simulink model "test"  (R2018b)
settings: Solver=FixedStepAuto  StartTime=0.0  StopTime=3  FixedStep=0.0001  RelTol=1e-3
settings Model: Creator=User  LastModifiedBy=User

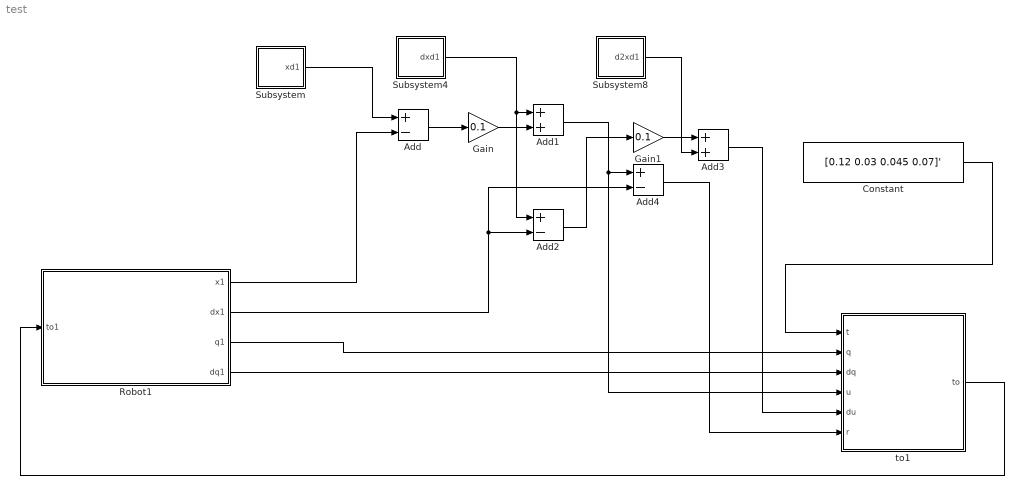
== system test ==
  Add : Sum  Inputs=+-
  Add1 : Sum
  Add2 : Sum  Inputs=+-
  Add3 : Sum
  Add4 : Sum  Inputs=+-
  Constant : Constant  Value=[0.12 0.03 0.045 0.07]'
  Gain : Gain  Gain=0.1
  Gain1 : Gain  Gain=0.1
  Robot1 : Subsystem
  Subsystem : Subsystem
  Subsystem4 : Subsystem
  Subsystem8 : Subsystem
  to1 : MATLAB Function  TreatAsAtomicUnit=on
  wires:
  to1/1(to) -> Robot1/1(to1)
  Add3/1 -> to1/5(du)
  Subsystem/1(xd1) -> Add/1
  Gain1/1 -> Add3/1
  Robot1/2(dx1) -> Add2/2, Add4/2
  Add1/1 -> to1/4(u), Add4/1
  Robot1/1(x1) -> Add/2
  Add2/1 -> Gain1/1
  Add/1 -> Gain/1
  Subsystem4/1(dxd1) -> Add2/1, Add1/1
  Add4/1 -> to1/6(r)
  Subsystem8/1(d2xd1) -> Add3/2
  Gain/1 -> Add1/2
  Robot1/3(q1) -> to1/2(q)
  Robot1/4(dq1) -> to1/3(dq)
  Constant/1 -> to1/1(t)

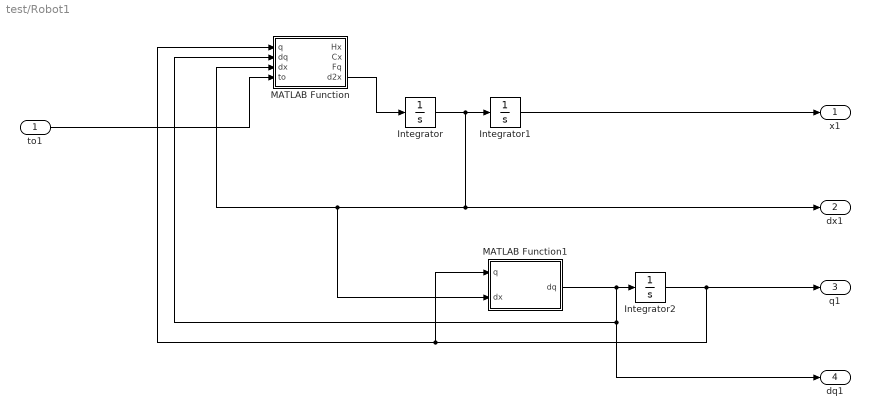
== system test/Robot1 ==
  to1 : Inport
  Integrator : Integrator  InitialCondition=[0;0]
  Integrator1 : Integrator  InitialCondition=[-3;-2]
  Integrator2 : Integrator  InitialCondition=[pi/6;pi/6]
  MATLAB Function : MATLAB Function  TreatAsAtomicUnit=on
  MATLAB Function1 : MATLAB Function  TreatAsAtomicUnit=on
  x1 : Outport
  dx1 : Outport  Port=2
  q1 : Outport  Port=3
  dq1 : Outport  Port=4
  wires:
  Integrator/1 -> MATLAB Function1/2(dx), MATLAB Function/3(dx), dx1/1, Integrator1/1
  MATLAB Function/4(d2x) -> Integrator/1
  to1/1 -> MATLAB Function/4(to)
  Integrator1/1 -> x1/1
  MATLAB Function1/1(dq) -> dq1/1, MATLAB Function/2(dq), Integrator2/1
  Integrator2/1 -> MATLAB Function/1(q), MATLAB Function1/1(q), q1/1

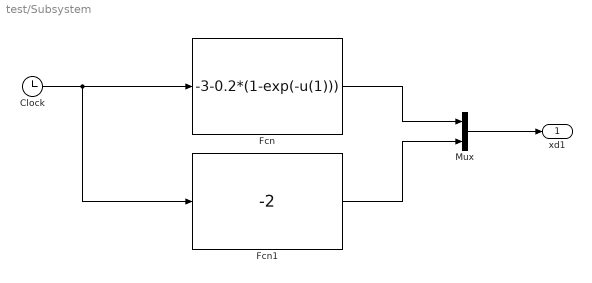
== system test/Subsystem ==
  Clock : Clock
  Fcn : Fcn  Expr=-3-0.2*(1-exp(-u(1)))
  Fcn1 : Fcn  Expr=-2
  Mux : Mux  Inputs=2
  xd1 : Outport
  wires:
  Clock/1 -> Fcn1/1, Fcn/1
  Fcn/1 -> Mux/1
  Fcn1/1 -> Mux/2
  Mux/1 -> xd1/1

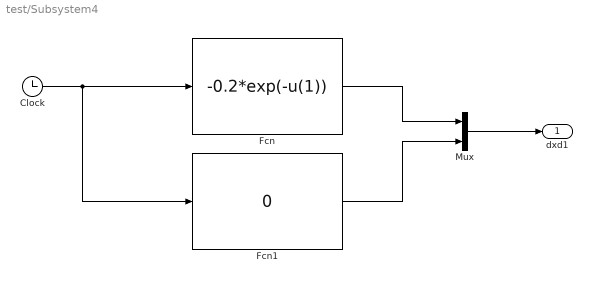
== system test/Subsystem4 ==
  Clock : Clock
  Fcn : Fcn  Expr=-0.2*exp(-u(1))
  Fcn1 : Fcn  Expr=0
  Mux : Mux  Inputs=2
  dxd1 : Outport
  wires:
  Mux/1 -> dxd1/1
  Fcn1/1 -> Mux/2
  Fcn/1 -> Mux/1
  Clock/1 -> Fcn/1, Fcn1/1

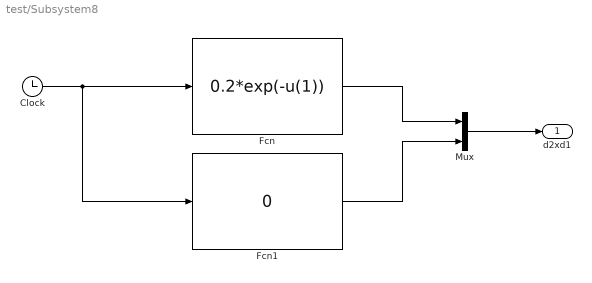
== system test/Subsystem8 ==
  Clock : Clock
  Fcn : Fcn  Expr=0.2*exp(-u(1))
  Fcn1 : Fcn  Expr=0
  Mux : Mux  Inputs=2
  d2xd1 : Outport
  wires:
  Clock/1 -> Fcn1/1, Fcn/1
  Fcn/1 -> Mux/1
  Fcn1/1 -> Mux/2
  Mux/1 -> d2xd1/1

== matlab function test/Robot1/MATLAB Function ==
  data: Hx output; Cx output; Fq output; q input; d2x output; dq input; dx input; to input
function [Hx,Cx,Fq,d2x] = fcn(q,dq,dx,to)
m1=1;
m2=1;
l1=0.3;
l2=0.3;
t1=1/3*m1*l1^2+m2*l1^2;
t2=1/3*m2*l2^2;
t3=1/2*m2*l1*l2;
t4=0.07;
q1=q(1);
q2=q(2);
Hq=[t1+t2+2*t3*cos(q2) t2+t3*cos(q2);
    t2+t3*cos(q2) t2];
dq1=dq(1);
dq2=dq(2);
Cq=[-dq2*t3*sin(q2) -(dq1+dq2)*t3*sin(q2);
    dq1*t3*sin(q2) 0];
Fq=[t4*dq1;t4*dq2];
J=[-0.3*sin(q1)-0.3*sin(q1+q2) -0.3*sin(q1+q2);
    0.3*cos(q1)+0.3*cos(q1+q2) 0.3*cos(q1+q2)];
dJ=[-0.3*dq1*cos(q1)-0.3*(dq1+dq2)*cos(q1+q2) -0.3*(dq1+dq2)*cos(q1+q2);
    -0.3*dq1*sin(q1)-0.3*(dq1+dq2)*sin(q1+q2) -0.3*(dq1+dq2)*sin(q1+q2)];
Hx=Hq*pinv(J);
Cx=Cq*pinv(J)-Hq*pinv(J)*dJ*pinv(J);
d2x=Hx\(to-Cx*dx-Fq);
end

== matlab function test/Robot1/MATLAB Function1 ==
  data: q input; dq output; dx input
function dq = fcn(q,dx)
q1=q(1);
q2=q(2);
J=[-0.3*sin(q1)-0.3*sin(q1+q2) -0.3*sin(q1+q2);
    0.3*cos(q1)+0.3*cos(q1+q2) 0.3*cos(q1+q2)];
dq=pinv(J)*dx;
end

== matlab function test/to1 ==
  data: t input; q input; dq input; u input; to output; du input; r input
function to = fcn(t,q,dq,u,du,r)
t1=t(1);
t2=t(2);
t3=t(3);
t4=t(4);
q1=q(1);
q2=q(2);
Hq=[t1+t2+2*t3*cos(q2) t2+t3*cos(q2);
    t2+t3*cos(q2) t2];
dq1=dq(1);
dq2=dq(2);
Cq=[-dq2*t3*sin(q2) -(dq1+dq2)*t3*sin(q2);
    dq1*t3*sin(q2) 0];
Fq=[t4*dq1;t4*dq2];
J=[-0.3*sin(q1)-0.3*sin(q1+q2) -0.3*sin(q1+q2);
    0.3*cos(q1)+0.3*cos(q1+q2) 0.3*cos(q1+q2)];
dJ=[-0.3*dq1*cos(q1)-0.3*(dq1+dq2)*cos(q1+q2) -0.3*(dq1+dq2)*cos(q1+q2);
    -0.3*dq1*sin(q1)-0.3*(dq1+dq2)*sin(q1+q2) -0.3*(dq1+dq2)*sin(q1+q2)];
Hx=Hq*pinv(J);
Cx=Cq*pinv(J)-Hq*pinv(J)*dJ*pinv(J);
to=Hx*du+Cx*u+Fq+1*r;
end
